simulink model "model4"  (R2022a)
settings: Solver=FixedStepAuto  StartTime=0.0  StopTime=20  FixedStep=1e-4  RelTol=1e-3
PreLoadFcn:
  | m = 3.600;     % kg
  | k = 400;    % N/m
  | b = 10;      % Ns/m
  | x0=1; %m
settings Model: Creator=Tsing  LastModifiedBy=Tsing

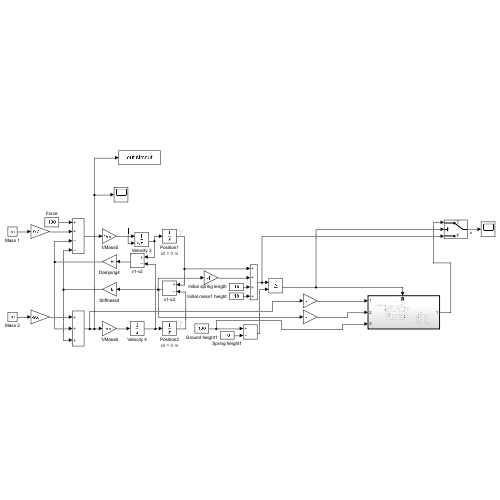
[thumbnail: Simulink's stored preview of the top-level diagram]
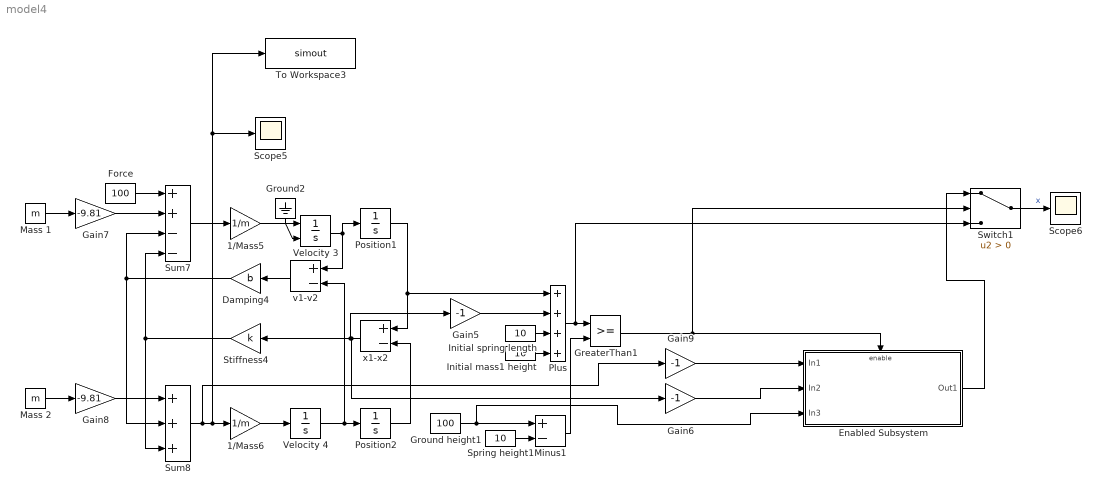
== system model4 ==
  1/Mass5 : Gain  Gain=1/m  SaturateOnIntegerOverflow=on  OutDataTypeStr=Inherit: Same as input  ParamDataTypeStr=Inherit: Same as input
  1/Mass6 : Gain  Gain=1/m  SaturateOnIntegerOverflow=on  OutDataTypeStr=Inherit: Same as input  ParamDataTypeStr=Inherit: Same as input
  Damping4 : Gain  Gain=b  SaturateOnIntegerOverflow=on  OutDataTypeStr=Inherit: Same as input  ParamDataTypeStr=Inherit: Same as input
  Enabled Subsystem : Subsystem  TreatAsAtomicUnit=on
  Force : Constant  Value=100
  Gain5 : Gain  Gain=-1
  Gain6 : Gain  Gain=-1
  Gain7 : Gain  Gain=-9.81
  Gain8 : Gain  Gain=-9.81
  Gain9 : Gain  Gain=-1
  GreaterThan1 : RelationalOperator  OutDataTypeStr=boolean  RndMeth=Simplest  InputSameDT=off
  Ground height1 : Constant  Value=100
  Ground2 : Ground
  Initial mass1 height : Constant  Value=10
  Initial spring length : Constant  Value=10
  Mass 1 : Constant  Value=m
  Mass 2 : Constant  Value=m
  Minus1 : Sum  Inputs=+-
  Plus : Sum  Inputs=++++
  Position1 : Integrator
      settings: AttributesFormatString=x0 = %<InitialCondition> m
  Position2 : Integrator
      settings: AttributesFormatString=x0 = %<InitialCondition> m
  Scope5 : Scope
  Scope6 : Scope
  Spring height1 : Constant  Value=10
  Stiffness4 : Gain  Gain=k  SaturateOnIntegerOverflow=on  OutDataTypeStr=Inherit: Same as input  ParamDataTypeStr=Inherit: Same as input
  Sum7 : Sum  Inputs=++--  InputSameDT=on  SaturateOnIntegerOverflow=on  OutDataTypeStr=Inherit: Same as first input
  Sum8 : Sum  Inputs=+++  InputSameDT=on  SaturateOnIntegerOverflow=on  OutDataTypeStr=Inherit: Same as first input
  Switch1 : Switch  Criteria=u2 > Threshold  SaturateOnIntegerOverflow=off  InputSameDT=off
  To Workspace3 : ToWorkspace  VariableName=simout  SaveFormat=Timeseries  SampleTime=-1
  Velocity 3 : Integrator  InitialConditionSource=external
  Velocity 4 : Integrator
  v1-v2 : Sum  Inputs=+-
  x1-x2 : Sum  Inputs=+-
  wires:
  Gain8/1 -> Sum8/1
  Mass 2/1 -> Gain8/1
  Sum8/1 -> Gain9/1, To Workspace3/1, Scope5/1, 1/Mass6/1
  Stiffness4/1 -> Sum7/4, Sum8/3
  Velocity 3/1 -> Position1/1, v1-v2/1
  Damping4/1 -> Sum8/2, Sum7/3
  Force/1 -> Sum7/1
  v1-v2/1 -> Damping4/1
  1/Mass5/1 -> Velocity 3/1
  Sum7/1 -> 1/Mass5/1
  Velocity 4/1 -> Position2/1, v1-v2/2
  Position1/1 -> Plus/1, x1-x2/1
  1/Mass6/1 -> Velocity 4/1
  Mass 1/1 -> Gain7/1
  Gain7/1 -> Sum7/2
  Position2/1 -> x1-x2/2
  x1-x2/1 -> Gain6/1, Stiffness4/1, Gain5/1
  Ground2/1 -> Velocity 3/2
  Spring height1/1 -> Minus1/2
  Ground height1/1 -> Enabled Subsystem/3(In3), Minus1/1
  Gain5/1 -> Plus/2
  Plus/1 -> Switch1/3, GreaterThan1/1
  Initial spring length/1 -> Plus/3
  Initial mass1 height/1 -> Plus/4
  Minus1/1 -> GreaterThan1/2
  GreaterThan1/1 -> Switch1/2, Enabled Subsystem/Enable
  Gain6/1 -> Enabled Subsystem/2(In2)
  Gain9/1 -> Enabled Subsystem/1(In1)
  Enabled Subsystem/1(Out1) -> Switch1/1
  Switch1/1 -> Scope6/1  "x"

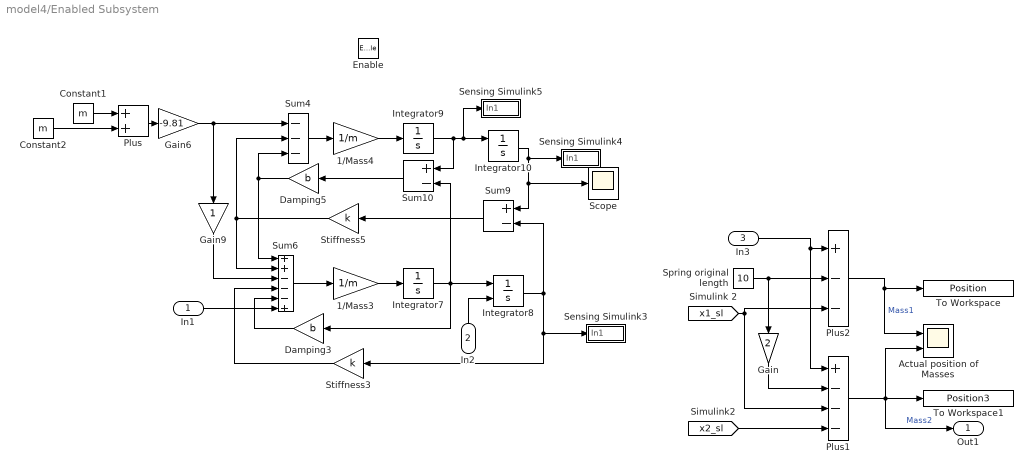
== system model4/Enabled Subsystem ==
  In1 : Inport
  In2 : Inport  Port=2
  In3 : Inport  Port=3
  Enable : EnablePort
  1/Mass3 : Gain  Gain=1/m  SaturateOnIntegerOverflow=on  OutDataTypeStr=Inherit: Same as input  ParamDataTypeStr=Inherit: Same as input
  1/Mass4 : Gain  Gain=1/m  SaturateOnIntegerOverflow=on  OutDataTypeStr=Inherit: Same as input  ParamDataTypeStr=Inherit: Same as input
  Actual position of Masses : Scope  NumInputPorts=2
  Constant1 : Constant  Value=m
  Constant2 : Constant  Value=m
  Damping3 : Gain  Gain=b  SaturateOnIntegerOverflow=on  OutDataTypeStr=Inherit: Same as input  ParamDataTypeStr=Inherit: Same as input
  Damping5 : Gain  Gain=b  SaturateOnIntegerOverflow=on  OutDataTypeStr=Inherit: Same as input  ParamDataTypeStr=Inherit: Same as input
  Gain : Gain  Gain=2
  Gain6 : Gain  Gain=-9.81
  Gain9 : Gain
  Integrator10 : Integrator  InitialConditionSource=external
      settings: AttributesFormatString=x0 = %<InitialCondition> m
  Integrator7 : Integrator
  Integrator8 : Integrator  InitialConditionSource=external
      settings: AttributesFormatString=x0 = %<InitialCondition> m
  Integrator9 : Integrator
  Plus : Sum
  Plus1 : Sum  Inputs=+---
  Plus2 : Sum  Inputs=+--
  Scope : Scope
  Sensing Simulink3 : Subsystem
      mask Display: disp('x1_sl')
  Sensing Simulink4 : Subsystem
      mask Display: disp('x2_sl')
  Sensing Simulink5 : Subsystem
      mask Display: disp('v2_sl')
  Spring original length : Constant  Value=10
  Stiffness3 : Gain  Gain=k  SaturateOnIntegerOverflow=on  OutDataTypeStr=Inherit: Same as input  ParamDataTypeStr=Inherit: Same as input
  Stiffness5 : Gain  Gain=k  SaturateOnIntegerOverflow=on  OutDataTypeStr=Inherit: Same as input  ParamDataTypeStr=Inherit: Same as input
  Sum10 : Sum  Inputs=+-  InputSameDT=on  SaturateOnIntegerOverflow=on  OutDataTypeStr=Inherit: Same as first input
  Sum4 : Sum  Inputs=---  InputSameDT=on  SaturateOnIntegerOverflow=on  OutDataTypeStr=Inherit: Same as first input
  Sum6 : Sum  Inputs=++---+  InputSameDT=on  SaturateOnIntegerOverflow=on  OutDataTypeStr=Inherit: Same as first input
  Sum9 : Sum  Inputs=+-  InputSameDT=on  SaturateOnIntegerOverflow=on  OutDataTypeStr=Inherit: Same as first input
  To Workspace : ToWorkspace  VariableName=Position  SaveFormat=Timeseries  SampleTime=-1
  To Workspace1 : ToWorkspace  VariableName=Position3  SaveFormat=Timeseries  SampleTime=-1
  Out1 : Outport
  wires:
  Damping3/1 -> Sum6/5
  Sum4/1 -> 1/Mass4/1
  Sum6/1 -> 1/Mass3/1
  Sum10/1 -> Damping5/1
  Integrator10/1 -> Sensing Simulink4/1(In1), Scope/1, Sum9/1
  Integrator9/1 -> Sensing Simulink5/1(In1), Integrator10/1, Sum10/1
  1/Mass4/1 -> Integrator9/1
  Stiffness5/1 -> Sum6/2, Sum4/2
  Sum9/1 -> Stiffness5/1
  1/Mass3/1 -> Integrator7/1
  Stiffness3/1 -> Sum6/4
  Damping5/1 -> Sum6/1, Sum4/3
  Integrator7/1 -> Sum10/2, Integrator8/1, Damping3/1
  Gain9/1 -> Sum6/3
  Gain6/1 -> Gain9/1, Sum4/1
  In2/1 -> Integrator8/2
  In1/1 -> Sum6/6
  Constant1/1 -> Plus/1
  Constant2/1 -> Plus/2
  Plus/1 -> Gain6/1
  [x1_sl] -> Plus1/3, Plus2/3
  Plus2/1 -> To Workspace/1, Actual position of Masses/1  "Mass1"
  In3/1 -> Plus1/1, Plus2/1
  Gain/1 -> Plus1/2
  Spring original length/1 -> Gain/1, Plus2/2
  [x2_sl] -> Plus1/4
  Plus1/1 -> Out1/1, To Workspace1/1, Actual position of Masses/2  "Mass2"
  Integrator8/1 -> Sum9/2, Sensing Simulink3/1(In1), Stiffness3/1

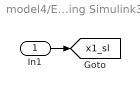
== system model4/Enabled Subsystem/Sensing Simulink3 ==
  In1 : Inport
  tag scope: x1_sl=global
  wires:
  In1/1 -> [x1_sl]

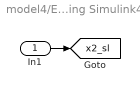
== system model4/Enabled Subsystem/Sensing Simulink4 ==
  In1 : Inport
  tag scope: x2_sl=global
  wires:
  In1/1 -> [x2_sl]

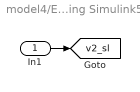
== system model4/Enabled Subsystem/Sensing Simulink5 ==
  In1 : Inport
  tag scope: v2_sl=global
  wires:
  In1/1 -> [v2_sl]
